simulink model "hyd_hyb_2_int_cont_Final"  (Simulink 8.2)
settings: Solver=ode4  StartTime=0  StopTime=3005  FixedStep=0.01  MaxStep=.4  RelTol=1e-8
InitFcn:
  | const_3_new
values from neighbouring files (symbols this model uses):
  Af = 6.3    [brk_enrg.m]    (also in brk_enrg_1.m)
  BSFC_906_205 = [3.5684 4.3466 5.1668 6.0769 6.988 7.8992 8.8104 9.7336 10.8548 11.9809 13.1112 14.2571 ... (663 elements, 39x17)]    [BSFC_map_906_205.mat]
  Cd = 0.55    [brk_enrg.m]    (also in brk_enrg_1.m)
  den = 1.202    [brk_enrg.m]    (also in brk_enrg_1.m)
  fr = 0.01    [brk_enrg.m]    (also in brk_enrg_1.m)
undefined symbols (not defined in the file or in its folder): clutchRise, down_spd_2, down_spd_3, down_spd_4, down_spd_c, Driving_Cycle, fuel_density, gearshift, I_wheel, Idle_spd_eng_906, M1_hydr, p_v_15, pmax_125, qv_125, Rw, sec_eng_sfc_map, T0, T1, T_max_906, T_min, TC_spd_ratio_max, teta_new_10, torque_convertor, Twait, up_spd_1, up_spd_2, up_spd_3, up_spd_c, v_p_10, v_p_15, v_p_5
libraries: neural x1742, fl_lib x43, nesl_utility x30, sdl_lib x14, simulink x4, simulink_need_slupdate x1
(part 24 of 26)

== system hyd_hyb_2_int_cont_Final/controller1/optimized controller/SOC upper 0.5/SOC upper 0.6/SOC upper 0.7/SOC upper 0.8/net_col_c_d_8_9/Layer 1/IW{1,1} ==
  "pd{1,1}" : Inport  PortDimensions=2
  "IW{1,1}(1,:)'" : Constant  Value=[5.2297082715673504;5.6273231620052648]
  "IW{1,1}(10,:)'" : Constant  Value=[5.3271967786741863;-5.5242837498455462]
  "IW{1,1}(11,:)'" : Constant  Value=[-5.7316192074747656;-5.0965749699765555]
  "IW{1,1}(12,:)'" : Constant  Value=[-6.7199302055662882;-3.6723493871487363]
  "IW{1,1}(13,:)'" : Constant  Value=[7.6310486911057183;-0.45691067438364946]
  "IW{1,1}(14,:)'" : Constant  Value=[-1.6156307363721207;-7.4985197467728266]
  "IW{1,1}(15,:)'" : Constant  Value=[7.6396721651827342;0.67767130428367428]
  "IW{1,1}(16,:)'" : Constant  Value=[-2.3794289636929844;-7.3027289928163359]
  "IW{1,1}(17,:)'" : Constant  Value=[7.609056298019194;0.96781732819446276]
  "IW{1,1}(18,:)'" : Constant  Value=[6.1297798419043019;4.6002468076239618]
  "IW{1,1}(19,:)'" : Constant  Value=[3.5487733537087367;6.8101240186103311]
  "IW{1,1}(2,:)'" : Constant  Value=[-1.7709080977346265;-7.442340947364527]
  "IW{1,1}(20,:)'" : Constant  Value=[4.6726604445306537;6.1099961278946511]
  "IW{1,1}(21,:)'" : Constant  Value=[3.625039631767633;-6.7490388004175426]
  "IW{1,1}(22,:)'" : Constant  Value=[2.3767648218081212;-7.2680324227364457]
  "IW{1,1}(23,:)'" : Constant  Value=[2.2051248172556823;7.3409202753957548]
  "IW{1,1}(24,:)'" : Constant  Value=[3.6000602042212226;6.7549906302868843]
  "IW{1,1}(25,:)'" : Constant  Value=[-6.6712233436411381;-3.6896842846457427]
  "IW{1,1}(26,:)'" : Constant  Value=[3.4549485140385632;-6.8529757203212176]
  "IW{1,1}(27,:)'" : Constant  Value=[3.9232555663050319;6.4420462296280734]
  "IW{1,1}(28,:)'" : Constant  Value=[0.80122508503254797;7.778785998543821]
  "IW{1,1}(29,:)'" : Constant  Value=[-3.0811819967324192;-6.8692043192527965]
  "IW{1,1}(3,:)'" : Constant  Value=[3.9369646308008228;6.5356049546767476]
  "IW{1,1}(30,:)'" : Constant  Value=[7.6499292380272141;1.3230721920060999]
  "IW{1,1}(4,:)'" : Constant  Value=[3.2253351379319164;6.9688557463217036]
  "IW{1,1}(5,:)'" : Constant  Value=[3.9082074631794095;6.5873222203975601]
  "IW{1,1}(6,:)'" : Constant  Value=[7.2679721529349646;2.4081951987663022]
  "IW{1,1}(7,:)'" : Constant  Value=[-7.5805190406682321;-1.0513803544595217]
  "IW{1,1}(8,:)'" : Constant  Value=[-3.9971056760000749;-6.5538153054232726]
  "IW{1,1}(9,:)'" : Constant  Value=[-5.1483853775004791;-5.691072714021133]
  Mux : Mux  Inputs=30
  dotprod{1..30} (30 alike) : neural/Weight Functions/dotprod
  "iz{1,1}" : Outport
  wires:
  Mux/1 -> "iz{1,1}"/1
  dotprod30/1 -> Mux/30
  "IW{1,1}(30,:)'"/1 -> dotprod30/1
  dotprod29/1 -> Mux/29
  "IW{1,1}(29,:)'"/1 -> dotprod29/1
  dotprod28/1 -> Mux/28
  "IW{1,1}(28,:)'"/1 -> dotprod28/1
  dotprod27/1 -> Mux/27
  "IW{1,1}(27,:)'"/1 -> dotprod27/1
  dotprod26/1 -> Mux/26
  "IW{1,1}(26,:)'"/1 -> dotprod26/1
  dotprod25/1 -> Mux/25
  "IW{1,1}(25,:)'"/1 -> dotprod25/1
  dotprod24/1 -> Mux/24
  "IW{1,1}(24,:)'"/1 -> dotprod24/1
  dotprod23/1 -> Mux/23
  "IW{1,1}(23,:)'"/1 -> dotprod23/1
  dotprod22/1 -> Mux/22
  "IW{1,1}(22,:)'"/1 -> dotprod22/1
  dotprod21/1 -> Mux/21
  "IW{1,1}(21,:)'"/1 -> dotprod21/1
  dotprod20/1 -> Mux/20
  "IW{1,1}(20,:)'"/1 -> dotprod20/1
  dotprod19/1 -> Mux/19
  "IW{1,1}(19,:)'"/1 -> dotprod19/1
  dotprod18/1 -> Mux/18
  "IW{1,1}(18,:)'"/1 -> dotprod18/1
  dotprod17/1 -> Mux/17
  "IW{1,1}(17,:)'"/1 -> dotprod17/1
  dotprod16/1 -> Mux/16
  "IW{1,1}(16,:)'"/1 -> dotprod16/1
  dotprod15/1 -> Mux/15
  "IW{1,1}(15,:)'"/1 -> dotprod15/1
  dotprod14/1 -> Mux/14
  "IW{1,1}(14,:)'"/1 -> dotprod14/1
  dotprod13/1 -> Mux/13
  "IW{1,1}(13,:)'"/1 -> dotprod13/1
  dotprod12/1 -> Mux/12
  "IW{1,1}(12,:)'"/1 -> dotprod12/1
  dotprod11/1 -> Mux/11
  "IW{1,1}(11,:)'"/1 -> dotprod11/1
  dotprod10/1 -> Mux/10
  "IW{1,1}(10,:)'"/1 -> dotprod10/1
  dotprod9/1 -> Mux/9
  "IW{1,1}(9,:)'"/1 -> dotprod9/1
  dotprod8/1 -> Mux/8
  "IW{1,1}(8,:)'"/1 -> dotprod8/1
  dotprod7/1 -> Mux/7
  "IW{1,1}(7,:)'"/1 -> dotprod7/1
  dotprod6/1 -> Mux/6
  "IW{1,1}(6,:)'"/1 -> dotprod6/1
  dotprod5/1 -> Mux/5
  "IW{1,1}(5,:)'"/1 -> dotprod5/1
  dotprod4/1 -> Mux/4
  "IW{1,1}(4,:)'"/1 -> dotprod4/1
  dotprod3/1 -> Mux/3
  "IW{1,1}(3,:)'"/1 -> dotprod3/1
  dotprod2/1 -> Mux/2
  "IW{1,1}(2,:)'"/1 -> dotprod2/1
  dotprod1/1 -> Mux/1
  "pd{1,1}"/1 -> dotprod30/2, dotprod29/2, dotprod28/2, dotprod27/2, dotprod26/2, dotprod25/2, dotprod24/2, dotprod23/2, dotprod22/2, dotprod21/2, dotprod20/2, dotprod19/2, dotprod18/2, dotprod17/2, dotprod16/2, dotprod15/2, dotprod14/2, dotprod13/2, dotprod12/2, dotprod11/2, dotprod10/2, dotprod9/2, dotprod8/2, dotprod7/2, dotprod6/2, dotprod5/2, dotprod4/2, dotprod3/2, dotprod2/2, dotprod1/2
  "IW{1,1}(1,:)'"/1 -> dotprod1/1

== system hyd_hyb_2_int_cont_Final/controller1/optimized controller/SOC upper 0.5/SOC upper 0.6/SOC upper 0.7/SOC upper 0.8/net_col_c_d_8_9/Layer 2/Delays 1 ==
  "p{2}" : Inport  PortDimensions=30
  mux : Mux  Inputs=1
  "pd{2,1}" : Outport
  wires:
  mux/1 -> "pd{2,1}"/1
  "p{2}"/1 -> mux/1

== system hyd_hyb_2_int_cont_Final/controller1/optimized controller/SOC upper 0.5/SOC upper 0.6/SOC upper 0.7/SOC upper 0.8/net_col_c_d_8_9/Layer 2/LW{2,1} ==
  "ad{2,1}" : Inport  PortDimensions=30
  "IW{2,1}(1,:)'" : Constant  Value=[-0.01337138047549283;-0.28095158446727192;-0.16503164756388625;-0.45784461439440827;-0.12950501000005665;0.18202533973662072;0.016691236840415163;-0.14736753510045073;-0.38808878997216451;0.30255086537017006;0.07200208164381916;0.56168796965376189;-0.45033706536037649;0.28342366252104456;-0.17290280054727319;0.099768076125372654;-0.30844788844149273;-0.48874450861518076;-0.095930800808782177;-0.085620551553359056;0.18719700480212248;0.20192166498704908;-0.39439281517504299;-0.1761066303970199;-0.27960083721330503;0.11415904568162979;0.33813666987772623;0.071160346914529549;-0.47467652276569738;0.53680426915168111]
  "IW{2,1}(10,:)'" : Constant  Value=[-0.12877936609158763;-0.47587728279057023;0.1877867845721852;-0.084215930155876292;-0.20839808710547195;-0.13666953154125866;0.35591088137150056;-0.14007053087915702;0.51663619503232094;0.44705116455638544;-0.20614768887343585;-0.30817662964547182;-0.11375336795447927;0.077503999867870141;-0.23895377418591321;-0.0041563317406688822;-0.35865623913112427;0.25243705879368766;-0.52549121959207545;-0.42448219196266607;0.39264365797558393;0.27932335621641147;-0.36925219355094963;0.31565733162137832;0.20118306741746081;-0.25536563672747148;0.14832240983231315;0.066442949083321184;-0.071777147677271794;-0.42005348211208249]
  "IW{2,1}(11,:)'" : Constant  Value=[0.42887485853389118;-0.48701290610635062;-0.018546953988905174;0.15083692230155854;-0.41499077481347629;-0.21432733820014618;-0.012686165000563823;0.42509965196917981;-0.035819058983909802;-0.57481434848859814;0.19499799217111058;0.15568572289966565;-0.18305925453768279;-0.021450482313967071;0.3661066323547566;0.046817351945665463;-0.35615081739053278;-0.0063144505914314491;0.47626161010990564;0.39519202026262112;0.38413528174445222;0.3325880859338356;0.31746601920344364;0.14701202960728005;0.31657075402271662;0.24974972097089457;0.37299354569369358;0.084383088674610862;0.12045514477163605;0.2263767581285841]
  "IW{2,1}(12,:)'" : Constant  Value=[-0.44785493325983433;0.29952879966428503;-0.3588623235389265;-0.18458233023437801;0.49357052273034574;-0.13165235315396617;-0.10119602952912031;-0.10260838617534325;-0.17126538459857643;-0.30572828086222886;0.29790579152294422;0.19409119242637829;0.21566604834666511;0.33688116278072733;0.24763106757804323;0.078656751347893794;-0.43440903548495796;-0.45551268819722224;0.38969396678151003;-0.22465887258290596;-0.23546967211109304;-0.29929980636648901;0.22900416155132622;0.092413420687598224;0.48574420859216094;-0.22374516140450662;-0.083901963510923591;0.30886163712497755;0.21685949872336133;0.061952852103937785]
  "IW{2,1}(13,:)'" : Constant  Value=[-0.31418908401409446;-0.26007649238943248;0.31954309252078866;-0.16814071124454713;-0.15763410114005866;-0.10401807888790811;-0.46102846038269585;0.25271545605528017;0.01007848864071678;-0.10314792312684756;0.1726838125829338;0.36931842608368276;0.3301744921687324;-0.3439717376221833;-0.2931194999336918;0.1567186462139446;0.028852670221030441;0.38095801360245324;-0.023951265973831792;-0.32362259435845647;0.1213573066251033;0.32671598025856813;-0.35992893349504707;0.39909077457579401;-0.31688075594830212;-0.26439448936765109;0.37925680164647591;0.40562213625379306;0.37358297909075522;-0.42747484886868137]
  "IW{2,1}(14,:)'" : Constant  Value=[0.44783714821849963;0.21410181269156028;0.0017982430301030691;-0.19465254425693904;-0.18537384377184216;0.56490668359860297;-0.14690102947081646;0.076463921210399077;-0.16204433876665503;0.36350674442905334;0.16992392694215283;0.12886172891572309;0.23470151490794303;-0.070262818563302507;0.15277790832690061;0.3242695891352198;-0.33513718132499548;0.02823581430237003;0.24246033346808166;-0.42088994103419702;-0.17302374067804713;0.0073299722701979375;0.12968092832442085;-0.17307640423438062;-0.47559342269963734;0.095925192804616047;-0.13976047960361213;0.1571766674662837;-0.50441234690224679;-0.52416221892977011]
  "IW{2,1}(15,:)'" : Constant  Value=[0.26248732607376118;0.49532186242617754;-0.50454391880052862;-0.327207659699144;-0.43642565615523787;-0.14607435486446912;0.40130138540730037;0.31215082826881574;0.25486274803394454;0.60973007559694337;0.33833680853014564;-0.52453062690783414;0.39088455441145586;0.078339660177359341;0.40661236585034116;-0.35387516353774034;0.0016044841618512832;0.16386400331983944;0.19567426275447886;-0.12013064942167608;-0.31208369937469305;-0.0072081351890981192;-0.089588039665270916;0.11873875205253952;-0.27994249441980767;-0.13508489135594531;0.17255143878117848;-0.22581311631817616;-0.12644715914540158;-0.087171365990115116]
  "IW{2,1}(16,:)'" : Constant  Value=[0.25849307971468227;-0.081086656772899016;-0.37114809548005617;0.25244334293572629;-0.43907061163932803;0.095907918504148287;0.00087443781706484985;0.0071769632098506201;-0.11045664266875481;0.27238467563200114;-0.48182337479969028;0.076178929039177418;-0.4290672354726795;0.1644471337080444;0.35539205679760533;-0.074161740982161509;-0.51362051686285326;-0.34302321993807111;0.093099865710912874;0.012061499461902237;-0.47011394461600625;0.082969559697853607;0.0082701803952539496;-0.18642695085794539;0.22494168965042269;0.38183906703217679;-0.2935199001717782;-0.42174419286554787;-0.096451078485828387;0.40643207224803157]
  "IW{2,1}(17,:)'" : Constant  Value=[-0.10985208829065081;0.20287921542786699;0.1385279804468377;-0.076191504229959808;-0.42580080975566248;0.14817967802448828;0.11089975305435197;0.42803122009154243;-0.37393350163109551;0.31184811677206176;0.19699926242620167;0.52047209393507121;0.23701277003839935;0.1655843122380026;0.30175170983751803;0.17624100149760077;0.16361599905038912;0.18855720151875785;-0.1980741670478727;-0.32967865622549619;-0.38664710435007577;-0.22380162289117694;-0.39779045097547805;0.42249107453632723;0.27410450945606801;0.34088477559968205;-0.047198280755287619;-0.21191075972781317;-0.25376453847567082;0.43719807532785637]
  "IW{2,1}(18,:)'" : Constant  Value=[0.36313113458044954;-0.45746696787424895;-0.34426640866793873;-0.32170606512569289;0.42057890979287332;-0.00181978915271525;0.1459272658151563;0.18519960726847709;-0.16106364805954584;-0.39963178414914424;-0.22157734573905408;0.32219734224641583;0.20062914162945403;-0.2545292998498267;0.35935237519802937;0.012926126328639867;0.45577500604689425;0.36355616414433117;0.43178218463070439;0.34368428016565061;-0.31142493031492391;0.0042379127935098272;0.13340593049872332;-0.08845582234622143;0.18892338612544646;0.15198499384350672;0.45809972028106005;0.0018658778608795163;0.15039472963027983;0.30140556377514649]
  "IW{2,1}(19,:)'" : Constant  Value=[-0.40024936770151809;-0.069990039918450486;-0.26846229603419031;-0.26796866623906085;0.14370094057409916;-0.13257757022718608;-0.14202670147981977;-0.11555052588655544;0.482513279982757;0.37540224984567433;0.045720880165311013;-0.34880970877999468;-0.084645593633637439;0.19675127038319284;0.3418468810673268;0.35818859368575673;0.28623906243260938;0.054468861071998345;-0.27715664772524884;0.53345353050796507;-0.28015882124595443;-0.22544662860211423;-0.18490067544779457;0.050219360778613213;-0.19199718879623881;0.35888889470113017;0.66475560302036896;0.36863432937801865;-0.18167039999527965;-0.24167470599647797]
  "IW{2,1}(2,:)'" : Constant  Value=[-0.17215825353448597;0.18276874727348558;0.41829311891188098;-0.38319630265046389;-0.3461732726853971;-0.34806187602749161;-0.031378949842030157;-0.053730269792174441;-0.31708091642943365;0.075250731893123868;0.077395970639861186;-0.43108799199953118;0.43648394912194644;0.23844679788483208;0.036329127847019096;-0.42482570873919556;0.12541331002972139;0.23262681737061769;-0.0884879688988226;-0.47080458980419865;-0.40740713775100956;0.29880858504804658;0.091433884817461827;0.27874073282329404;0.10002048156338145;0.31048702807117606;-0.40704393944417033;-0.32206176394111002;-0.20514600682087514;0.024424815321697994]
  "IW{2,1}(20,:)'" : Constant  Value=[-0.38223287733513139;-0.11651569769184145;-0.23275015969836332;-0.45779281349779999;0.18066173843842123;0.023085666550045913;-0.40820570256541683;0.33916201754344916;-0.11266284908532383;-0.16903683306578501;-0.28648097306394582;-0.43083926662310867;-0.46970003759028961;0.41457450668029128;0.31816631920923794;-0.071101200865994502;-0.37495314507762695;-0.33674199314348485;0.25952681605999778;0.23489594693223437;-0.10125495737454836;0.2101344479027816;0.37005895040677289;0.30587065555411441;0.063143632678687708;0.28455037362744107;0.36363792391389332;0.20145534806805193;0.41971752395757178;-0.079369589634068052]
  "IW{2,1}(21,:)'" : Constant  Value=[-0.44587557795505756;0.32740561952944419;0.38242609904269403;0.37430642058075175;-0.16068302641590787;0.41726742666478989;0.14942045232082238;-0.1621253464371438;-0.32622675546004437;-0.32116770641464681;-0.36557171156205387;0.36502044171332571;0.27334850926184612;-0.30009388144256499;0.42802284457067563;0.14466585140373142;-0.060258875798323314;-0.41742951301170372;0.23808745747733381;0.18585314943781042;0.053722779449327886;0.054664173200892778;0.15483250040667215;0.20287679547981879;0.38366880349904847;0.20457898436260571;0.16469380057399624;-0.29360888772298599;-0.42080913578445506;0.046179995566540122]
  "IW{2,1}(22,:)'" : Constant  Value=[0.21636058009297521;-0.048628316899150946;0.22400575098582581;-0.16240083162601937;-0.27981474426276076;-0.07157564563365007;-0.2350472772516605;0.25118377072926423;0.35912589234946107;0.076186507209085083;0.22161975625797509;0.15702030333433434;-0.43095922425841232;-0.4152102657603447;-0.43862743602039422;-0.011235991663650854;-0.13312099176855877;0.30415086968488675;-0.31121424612693388;-0.33791185979529931;0.23077084628641112;0.28344905486157063;-0.53611342527279215;-0.2015566312576936;-0.21547089435873504;0.39763390440517432;-0.16950914148141671;-0.53712866466562004;-0.17652712530811226;-0.3427999056643391]
  "IW{2,1}(23,:)'" : Constant  Value=[-0.35280675392156435;-0.3010673935021328;0.41608246319314468;-0.33849225058032895;0.22991102374993189;0.32333061389512163;-0.084652038040488695;-0.19154035498842203;0.29772109061750851;0.30170392247270678;0.3581450372963832;0.065280684788798629;0.2767167597231473;-0.20308742181054668;-0.44195273570782612;-0.3732427508820168;-0.22105404763754652;-0.10469193681428836;0.4311958385750429;-0.065795408024307694;-0.15641781925152709;-0.23510602786800178;0.30249970235825796;0.22936052939810028;-0.39549613705286923;-0.3361265711189701;-0.16519320632831874;-0.26305919328914285;-0.32180519874075603;0.35878969944792594]
  "IW{2,1}(24,:)'" : Constant  Value=[-0.39954818514968038;-0.38584858299109431;-0.07541952652740487;-0.20450550652773936;-0.0093294507875483438;-0.52669564687724446;0.38351113947591614;0.49383839797094709;-0.18039270622145775;-0.29122897578217299;-0.35920060664312431;0.14092558998120627;0.1980150762491856;-0.047907822931633183;0.34783764602231987;-0.64517520829618358;-0.2143138418484537;0.081914435692262089;-0.29039775640602383;0.30932947623581064;-0.38977163386739161;0.2512912654662966;0.2307235760701683;-0.043076335891067401;0.23872064932855175;-0.33349036996482201;0.069572227976522599;-0.55478052347580242;0.57110817405267611;-0.093336083351195434]
  "IW{2,1}(25,:)'" : Constant  Value=[-0.36763713801641079;0.34825941736863519;0.42454373002714263;0.28313626181003215;0.10629586035838771;0.34705077686493213;-0.17379537371878279;0.3939219596097247;-0.35511501178728516;0.30538906314992975;-0.33086578883535178;0.27933314751540111;0.063771123735152049;0.078970554978038288;0.37006133520646994;0.11259355433337212;0.35343274160777882;-0.28812607166442028;0.16935010416359675;-0.36502314661876956;0.4617288314214128;-0.11547186509230255;0.046403829322165462;-0.22169916114863508;0.38623192167903392;0.41959430731705616;0.32414954279425734;-0.075205581037819505;0.15790599393630386;0.37414078448769206]
  "IW{2,1}(26,:)'" : Constant  Value=[0.52573288749680702;0.40034099811987017;-0.26614507154943695;-0.17639794797590561;-0.16509663241579434;-0.22664989154653412;0.065061930792583406;0.11228960496979679;-0.01586496866196091;-0.16684352947742317;0.20796323056056001;0.54615267784543953;-0.23128711278068634;0.15776886108586116;-0.44292144158175684;-0.097466048631904056;-0.31799965938536556;-0.26010448981072015;-0.17307094257448311;-0.18913055968361217;0.017575167502147836;-0.041939063149283952;0.43861409427711379;0.013801766692959388;-0.22718167304398099;-0.28560079969741436;0.38903185419408859;-0.50312163030440182;0.31408250210754701;0.37665101738300977]
  "IW{2,1}(27,:)'" : Constant  Value=[0.33171371527714699;0.16094842839367779;-0.43394200050156834;0.22369320776146284;0.29166008248048902;0.27252752447324446;0.36954493029020469;0.51971771989356952;0.18853850210773501;-0.38736530853307249;0.20057642766429876;-0.16322009210808275;-0.46668975066387747;0.12815905353447782;0.41584758680762668;-0.15897244145771519;0.0075665170752451686;0.29045355417878171;-0.30879748700008658;-0.52223839170982966;0.200570563279833;0.10492517778771469;-0.28682697922584538;-0.2809972048979455;-0.082528614229641278;-0.099363495498231716;-0.18145867697150497;0.31196931752430912;-0.24493689473639332;-0.052841565698375143]
  "IW{2,1}(28,:)'" : Constant  Value=[0.46352443075216065;-0.16020812737041185;0.11617096384756628;0.084739151585717598;-0.005397449191996649;0.33740212936135172;0.15352153436759949;-0.37872991144121126;0.44672032463976857;-0.21011996332232627;-0.24880878776884566;0.43728779774751936;-0.33719912988739931;-0.23352942228598422;-0.15288243110157007;-0.16213244976095589;-0.14952286234315387;0.087128460914169911;-0.33304589754894048;0.58262554536069033;-0.31376856708129131;0.10334800924732476;-0.3263613131405364;0.18621928005460742;0.26070946741513235;0.37499179915623981;0.32227956879442249;0.16628976408850452;0.36124072198989432;0.30241654834024695]
  "IW{2,1}(29,:)'" : Constant  Value=[-0.032135656874180109;0.07782054152925845;0.0040382908002594654;0.29595481169961307;-0.49719562651437715;0.045881703436677357;-0.13674251619170574;-0.3651454127633163;0.37753762710669941;0.015070789295483392;0.38137989535205796;-0.44740028262003767;-0.35796445021792894;0.16308738337540649;0.40614755086184079;0.25417112757858445;0.14995071389086537;0.15778841738949609;-0.42509024816716812;-0.35724418187985457;-0.34910295369786914;0.15678899210307395;0.3638484253106663;-0.47125321250771501;0.091804607727718243;-0.16270328791294161;-0.37000259210045022;-0.38839262070853597;0.010645208949013392;0.28440502208264956]
  "IW{2,1}(3,:)'" : Constant  Value=[0.49589068496557848;-0.099790505715858333;0.19907432476762735;-0.15103188678785306;-0.12154785305984357;0.019985691440159107;0.42440771674479172;-0.11330245780436633;-0.098572061777852077;0.14407479352187666;-0.36614585708981523;-0.31411433621055823;-0.19653030232966009;-0.093984011944081;-0.2498301487471056;0.17850968751630122;0.23507025422671757;0.25555893873650432;0.47760052403438508;0.49303832040789719;0.18479749666760689;0.54780287375494663;-0.024168247943590095;-0.049713587351482194;-0.052804916716366966;-0.5531654257761387;-0.042124019466908975;0.23243801723715074;0.085949288304206062;0.50513626708486281]
  "IW{2,1}(30,:)'" : Constant  Value=[-0.049539611263283823;-0.21050388986124069;0.36854535771673841;0.35646862647244404;-0.12945675563556919;-0.058142221328256034;-0.35472560017380977;-0.22294006236398664;0.36491124821386312;-0.37704006333052648;0.15195308817791128;-0.23083299918527303;-0.49723252321599637;-0.15776468530387094;0.29131945332116121;-0.4919654897132395;-0.22849123180584444;-0.40567867617927333;0.16937452809726758;0.2277476637397505;-0.29036301627548894;-0.34298893911860306;0.28254362300492175;0.13584255131354611;-0.3009081560459887;-0.007315560129343153;0.22990789594098793;0.35945961483827538;-0.321277457766523;0.34274055153256355]
  "IW{2,1}(31,:)'" : Constant  Value=[-0.16132811963159346;-0.05062360531953828;-0.37672644648510456;0.067530469560452125;-0.12358081954064448;-0.3073367745663908;-0.49757470974951779;-0.035677851183680019;-0.23072579152072942;0.31870379457497505;-0.20214077549455436;-0.28618563654097257;-0.096067278036762557;0.46270416622365801;0.46748405885863137;-0.16688562101496926;-0.34790847357964105;0.035411119946928866;-0.30970842080054145;0.4166094000270677;-0.094592761732787842;-0.17090119044849839;0.4591296289596577;-0.22987076579145688;0.049029546631407489;0.20057854380811307;-0.43708930157420478;0.16332184135462674;-0.24965469474306659;-0.4399386232667104]
  "IW{2,1}(32,:)'" : Constant  Value=[-0.10960003224877882;-0.43018847706807839;0.51600023685217689;-0.54680117952894602;-0.20074674176317087;0.24530234075343244;0.56756028812749448;0.43984120340234445;-0.36682999450401838;-0.31524978946179366;-0.44416640904854154;0.042777969880379386;0.19299135061331887;0.0085978860053103744;0.10492200544185569;0.013562235105007201;0.0067268931617746946;0.41604794698378683;0.061651283693760474;0.080303691432675309;0.13375639018360874;0.45708453079471084;-0.01589778034387028;0.16772634511867013;-0.10718683962112731;-0.073499940581839965;-0.11748968833344255;0.31257620440872097;-0.44650296770344555;-0.24283220910008219]
  "IW{2,1}(33,:)'" : Constant  Value=[0.44309314489416107;-0.19407213446434163;0.29095073825095674;0.41485201784327885;0.1997842537710604;-0.048894504535411817;0.1483106326562916;-0.030054084121407171;0.47059399352590481;-0.039251170687077938;-0.27095604380657484;-0.018301125390313259;-0.22525355966166052;0.18209500442869841;0.044678593285385641;0.41350426852397471;-0.42466178548153199;0.25563245497413783;-0.31647268041785948;-0.29381900366836344;-0.17082615688039818;-0.36473588127055045;0.54568761453444214;0.33891407074749547;0.432181267674211;0.014859918413714958;-0.22028136579632701;-0.0023456653160113861;0.51817674045931039;0.15125382899578843]
  "IW{2,1}(34,:)'" : Constant  Value=[0.32921363085196775;0.05562151583568159;-0.35034077400782743;0.25012478306330471;-0.13017943304241886;0.3433967030031615;0.29597295356986908;-0.210137558377266;0.41214383333754445;-0.21845816248736727;-0.29589408914469384;-0.3303403345752412;-0.2198668799882193;0.37805878861588205;-0.344667271778625;-0.1090280719538483;-0.096313448723471529;-0.26228271369138578;-0.40027321789097597;0.42086673720411261;-0.12071877246969784;0.046042297244496162;0.34950811699336254;0.47448331798639004;-0.16177072531830192;-0.33548521113654028;0.36399399605948313;0.4851527629749392;-0.42119637494713347;0.20255457814559419]
  "IW{2,1}(35,:)'" : Constant  Value=[-0.095304181568827057;0.2411861797336044;0.38093256060531172;-0.38482836195195164;-0.20955113698622385;-0.22805076013641554;0.29720949253117951;-0.16063823229995752;0.35958482194483726;-0.026755554233294628;0.15727655096687126;-0.1728035938490618;0.057094024908256977;0.01526672348094682;0.39237780589301491;0.45867076500022103;0.5581416472088867;0.42758505831315785;-0.030390232255899031;0.073219907667348982;0.16574749841546035;-0.0048104100066032243;0.1788932676861425;-0.35448965871809562;0.55469357014382281;-0.56191267035479397;0.1111925277258709;0.13606601060132853;-0.12582903254498432;-0.21658224463438697]
  "IW{2,1}(36,:)'" : Constant  Value=[-0.19128044878020015;-0.10994557683321811;-0.49575647432059594;-0.52362892158725849;-0.27280257170184113;0.068185085406951021;-0.19714897729908581;0.35444168343320737;-0.092621955922172955;-0.49572669586490964;0.57202494584954167;0.3278340339248309;-0.50884757125464375;-0.27301784455461925;0.14507662918967204;-0.27534742727516476;0.025149085320547541;-0.20293411172988976;0.1312925370460527;-0.19007693669979023;0.052619675958508853;-0.44475110339492713;0.045983399704365359;-0.14992425385717129;-0.41466020405617054;0.41639532250839117;0.29279888946762456;0.43706899341141237;-0.23911442125931215;-0.46610174086974565]
  "IW{2,1}(37,:)'" : Constant  Value=[0.23372418297866729;0.053635735470619075;0.42145802794127607;0.47036015295360345;-0.016586558717063344;-0.32643857468136195;-0.28371518742311513;0.09803946857466575;0.32359913792801265;-0.13943681923849011;0.2984112743599634;0.38504949535570676;-0.46419048466057555;0.35449184941958323;-0.45034003692534913;0.007248493685549617;0.41318157774100067;0.13694508099330388;-0.14105313192375307;0.31040845146413543;-0.42577850854320587;-0.39614305903626607;0.036802040775937885;-0.28240306172789981;0.34335509546632009;-0.11303859296920049;0.083892521426806671;-0.33789689302338088;-0.099731721936320822;0.11018262070533315]
  "IW{2,1}(38,:)'" : Constant  Value=[0.28099261784900359;0.3193879716122931;0.42728098016589555;0.31657025567995195;0.45108980800229204;0.22831118471030978;-0.13386410394994516;-0.068164403512579047;-0.34508904764661219;0.3876237504787986;-0.00044624195542457989;0.16554559092654872;0.23283464736276793;0.36393882914020215;0.36640897303212555;0.013768397221129993;0.41075269006827014;0.13356036927354209;-0.28997312141977305;0.073751840513592556;-0.33401994822798786;0.30757744605086701;-0.40284577898625334;0.072202088999151884;-0.4171213915393871;-0.12573436898940651;0.0068675004406296737;-0.38796886773544875;-0.38360973643403273;-0.19326434765954589]
  "IW{2,1}(39,:)'" : Constant  Value=[-0.32757754884726292;-0.079798672827026032;-0.43617646227829049;0.092408938920207837;-0.18053063251777915;-0.45222968309602551;-0.033681065820181343;0.09233311332115815;0.36045287074028109;0.18767183113811103;0.41516942119227845;-0.30722382070363563;-0.4254720917525931;0.19297915653605641;0.39811802646308864;-0.33799835929339955;0.26481767727562383;-0.07583865459147382;0.052761978622893169;-0.41484250073497653;0.46060901006667493;-0.17291735604678432;0.23866041452916714;-0.43666657192707836;0.11272059076303981;0.4282678664838101;-0.2013228359819747;-0.33541571927699376;-0.23190326147435741;-0.28162051653985287]
  "IW{2,1}(4,:)'" : Constant  Value=[-0.1033101588955887;0.19723778811968759;-0.050334669662173023;-0.40401992912827744;-0.37203771263235458;-0.070862259775875375;0.17265165146385897;0.45120564616098313;-0.30033568297024749;-0.095377549075230869;-0.22461822793898964;-0.033382595978892565;0.051799243492291397;-0.1920663496419826;0.44772114437237798;-0.20290977837278368;-0.45208788758642804;0.0041700277232766952;-0.32896667827504528;-0.44277943415629684;-0.16884441208067191;-0.15018007843166128;-0.35614725409236908;0.061998033725852567;0.4472656016464307;0.42130255096292724;0.3946318694739227;0.30959329779026257;0.40045309040204125;0.030639466028702874]
  "IW{2,1}(40,:)'" : Constant  Value=[0.15046878531670518;-0.30672503393827633;0.22411832901650924;0.13509624688313518;-0.34571378382937207;0.066805973069938129;-0.27876460666036157;0.46102713903022396;-0.25291888010956842;0.10868076501566555;0.25246055232063602;0.17258627267115154;0.24430979399509889;0.089281500966414032;0.33788350015495006;0.017431540868197235;0.44545920044149367;-0.39497816501439265;-0.1144001399018838;0.31038743348810499;0.19121596309155492;0.0080988710505405168;-0.21618039945702153;0.46885068859535084;-0.29164901874853866;0.4655136896867117;-0.32013789260363212;0.0074623519291403704;0.43115342101542409;0.45197306786998637]
  "IW{2,1}(5,:)'" : Constant  Value=[0.035084508806841483;-0.22309699429840305;0.31847817403339324;0.075239299837429094;-0.39273716495940869;-0.094184962576489561;-0.033172473093734313;0.14606226763656099;0.0930816854706535;-0.43223819820786291;-0.23023870285717199;-0.46103740043144392;0.33041911494577042;-0.0038860200166226889;0.27567793872830865;-0.43963490714533127;-0.21732527501532825;-0.15757997026674148;-0.40296802299020507;0.11323597593401873;0.39098520712327417;0.18849632930202284;0.40028433685325543;0.43204735194293514;-0.45141872795683829;0.27813157442337627;0.47632451016231397;-0.33572133057980974;-0.40728861097546198;0.1821846099423006]
  "IW{2,1}(6,:)'" : Constant  Value=[0.061689139330504961;0.47503152929291875;-0.23508033613305421;0.032368945162306394;0.16141041481701496;0.49898938245359176;0.14620097648708399;-0.12998956897472833;0.26981476837151974;-0.14479328909394082;0.37118496890031782;0.12247390959540533;0.60256439895707281;0.2732823395600209;0.27706091645880071;-0.24813973636499584;-0.37723372169828717;0.031282335938951286;-0.16495803738202042;0.19539376318442231;0.22644918670236683;-0.018018305447286539;-0.43812820063951885;-0.039801640209229799;-0.42404653533843284;-0.1150955597325749;-0.20902331603204333;-0.44516744448648798;-0.3109361036481984;0.26913433021580241]
  "IW{2,1}(7,:)'" : Constant  Value=[0.37549651462473788;0.20016705528187573;-0.20630460323959807;0.18473032347994298;0.30139670694994908;-0.32882887048936998;0.034469628218871291;0.062888103668764933;-0.42373630734630624;-0.2026860520356113;0.45737971815981304;0.27491666965410916;-0.28601117658794017;-0.22258265729116961;0.44516348538260619;-0.20008300765465481;-0.17685032666878078;0.095713508905817923;-0.44745074901871257;-0.29721183143062513;-0.38889753890692025;0.082991607687713173;0.41465796413739264;0.27770788778360733;0.33246673320645831;0.13176507381700622;0.06853705330887773;-0.16090863406100647;-0.49708819367776025;0.12290505058921722]
  "IW{2,1}(8,:)'" : Constant  Value=[0.12895028439581618;-0.0010177320513798951;-0.13629719225032341;-0.45165414971870965;0.44758354424095537;-0.40686506362381736;-0.26955513540494597;-0.44442908676720144;0.18485782026388561;0.15019243336851781;0.19933474473485449;-0.014863908837363507;0.30239437021814047;-0.10137091311622576;-0.1207035912245293;0.11605085175893905;-0.30164213974845211;-0.22280866074564185;-0.19505302686720979;0.23219967640280631;-0.4698159463542313;0.081861226183918875;0.12039789510468725;0.42129998556648551;-0.35156531504035232;-0.18789588586684891;0.1871546109807222;-0.44837952067230014;0.44141433402483332;0.32048534399380912]
  "IW{2,1}(9,:)'" : Constant  Value=[0.093949687257767367;0.28291752064807069;-0.37801438477294214;0.38400904730423085;-0.40277799298334105;-0.17893428464271008;-0.12545782038178244;-0.30965344807437317;-0.31078103980540567;-0.07348897089833635;0.37256928599431838;-0.16735615211311111;0.27169321886679421;0.32805839937562098;-0.0051331807985233752;-0.3253297505738878;0.3002643609297499;-0.23585187783813935;-0.52318354831089209;-0.28846738635763242;-0.26888748279035318;-0.10928234646665251;-0.56936096690595006;0.19762261966641231;0.014523717854880866;-0.196534962868882;0.45761981386523953;0.090252012488458586;0.12102086920512532;-0.29466926370148916]
  Mux : Mux  Inputs=40
  dotprod{1..40} (40 alike) : neural/Weight Functions/dotprod
  "lz{2,1}" : Outport
  wires:
  Mux/1 -> "lz{2,1}"/1
  dotprod40/1 -> Mux/40
  "IW{2,1}(40,:)'"/1 -> dotprod40/1
  dotprod39/1 -> Mux/39
  "IW{2,1}(39,:)'"/1 -> dotprod39/1
  dotprod38/1 -> Mux/38
  "IW{2,1}(38,:)'"/1 -> dotprod38/1
  dotprod37/1 -> Mux/37
  "IW{2,1}(37,:)'"/1 -> dotprod37/1
  dotprod36/1 -> Mux/36
  "IW{2,1}(36,:)'"/1 -> dotprod36/1
  dotprod35/1 -> Mux/35
  "IW{2,1}(35,:)'"/1 -> dotprod35/1
  dotprod34/1 -> Mux/34
  "IW{2,1}(34,:)'"/1 -> dotprod34/1
  dotprod33/1 -> Mux/33
  "IW{2,1}(33,:)'"/1 -> dotprod33/1
  dotprod32/1 -> Mux/32
  "IW{2,1}(32,:)'"/1 -> dotprod32/1
  dotprod31/1 -> Mux/31
  "IW{2,1}(31,:)'"/1 -> dotprod31/1
  dotprod30/1 -> Mux/30
  "IW{2,1}(30,:)'"/1 -> dotprod30/1
  dotprod29/1 -> Mux/29
  "IW{2,1}(29,:)'"/1 -> dotprod29/1
  dotprod28/1 -> Mux/28
  "IW{2,1}(28,:)'"/1 -> dotprod28/1
  dotprod27/1 -> Mux/27
  "IW{2,1}(27,:)'"/1 -> dotprod27/1
  dotprod26/1 -> Mux/26
  "IW{2,1}(26,:)'"/1 -> dotprod26/1
  dotprod25/1 -> Mux/25
  "IW{2,1}(25,:)'"/1 -> dotprod25/1
  dotprod24/1 -> Mux/24
  "IW{2,1}(24,:)'"/1 -> dotprod24/1
  dotprod23/1 -> Mux/23
  "IW{2,1}(23,:)'"/1 -> dotprod23/1
  dotprod22/1 -> Mux/22
  "IW{2,1}(22,:)'"/1 -> dotprod22/1
  dotprod21/1 -> Mux/21
  "IW{2,1}(21,:)'"/1 -> dotprod21/1
  dotprod20/1 -> Mux/20
  "IW{2,1}(20,:)'"/1 -> dotprod20/1
  dotprod19/1 -> Mux/19
  "IW{2,1}(19,:)'"/1 -> dotprod19/1
  dotprod18/1 -> Mux/18
  "IW{2,1}(18,:)'"/1 -> dotprod18/1
  dotprod17/1 -> Mux/17
  "IW{2,1}(17,:)'"/1 -> dotprod17/1
  dotprod16/1 -> Mux/16
  "IW{2,1}(16,:)'"/1 -> dotprod16/1
  dotprod15/1 -> Mux/15
  "IW{2,1}(15,:)'"/1 -> dotprod15/1
  dotprod14/1 -> Mux/14
  "IW{2,1}(14,:)'"/1 -> dotprod14/1
  dotprod13/1 -> Mux/13
  "IW{2,1}(13,:)'"/1 -> dotprod13/1
  dotprod12/1 -> Mux/12
  "IW{2,1}(12,:)'"/1 -> dotprod12/1
  dotprod11/1 -> Mux/11
  "IW{2,1}(11,:)'"/1 -> dotprod11/1
  dotprod10/1 -> Mux/10
  "IW{2,1}(10,:)'"/1 -> dotprod10/1
  dotprod9/1 -> Mux/9
  "IW{2,1}(9,:)'"/1 -> dotprod9/1
  dotprod8/1 -> Mux/8
  "IW{2,1}(8,:)'"/1 -> dotprod8/1
  dotprod7/1 -> Mux/7
  "IW{2,1}(7,:)'"/1 -> dotprod7/1
  dotprod6/1 -> Mux/6
  "IW{2,1}(6,:)'"/1 -> dotprod6/1
  dotprod5/1 -> Mux/5
  "IW{2,1}(5,:)'"/1 -> dotprod5/1
  dotprod4/1 -> Mux/4
  "IW{2,1}(4,:)'"/1 -> dotprod4/1
  dotprod3/1 -> Mux/3
  "IW{2,1}(3,:)'"/1 -> dotprod3/1
  dotprod2/1 -> Mux/2
  "IW{2,1}(2,:)'"/1 -> dotprod2/1
  dotprod1/1 -> Mux/1
  "ad{2,1}"/1 -> dotprod40/2, dotprod39/2, dotprod38/2, dotprod37/2, dotprod36/2, dotprod35/2, dotprod34/2, dotprod33/2, dotprod32/2, dotprod31/2, dotprod30/2, dotprod29/2, dotprod28/2, dotprod27/2, dotprod26/2, dotprod25/2, dotprod24/2, dotprod23/2, dotprod22/2, dotprod21/2, dotprod20/2, dotprod19/2, dotprod18/2, dotprod17/2, dotprod16/2, dotprod15/2, dotprod14/2, dotprod13/2, dotprod12/2, dotprod11/2, dotprod10/2, dotprod9/2, dotprod8/2, dotprod7/2, dotprod6/2, dotprod5/2, dotprod4/2, dotprod3/2, dotprod2/2, dotprod1/2
  "IW{2,1}(1,:)'"/1 -> dotprod1/1

== system hyd_hyb_2_int_cont_Final/controller1/optimized controller/SOC upper 0.5/SOC upper 0.6/SOC upper 0.7/SOC upper 0.8/net_col_c_d_8_9/Layer 3/Delays 1 ==
  "p{3}" : Inport  PortDimensions=40
  mux : Mux  Inputs=1
  "pd{3,2}" : Outport
  wires:
  mux/1 -> "pd{3,2}"/1
  "p{3}"/1 -> mux/1

== system hyd_hyb_2_int_cont_Final/controller1/optimized controller/SOC upper 0.5/SOC upper 0.6/SOC upper 0.7/SOC upper 0.8/net_col_c_d_8_9/Layer 3/LW{3,2} ==
  "ad{3,2}" : Inport  PortDimensions=40
  "IW{3,2}(1,:)'" : Constant  Value=[-0.69911497170846826;-0.84968559473564587;0.93001417164508637;0.018202841756782048;0.76378491660665193;0.84914790052554001;-0.22866747930600972;-0.70988610283860432;-0.37369799840908985;-0.77413605436519262;-0.63667272785630602;-0.13934641013435334;-0.41405897236010791;-0.50325625051054479;1.1492329270259298;0.61933422714591557;-0.7657963304111004;-0.038376686711376902;-0.66711670279845703;-0.76082072180098936;0.17440556360546713;0.089970343924166307;-0.21834942423226728;-1.0721888491060685;-0.78210940401126205;-0.45017112518459645;0.1892988776329437;-1.0423381607025282;0.56208969326132274;-0.38660183925036612;-0.57815958836389136;-0.7345342692876411;0.93555241069437889;0.84386167904683085;0.18599157668689836;0.94138927521719373;0.11694894528843508;-0.05118440700807754;-0.51667371394154937;-0.24648808072009776]
  Mux : Mux  Inputs=1
  dotprod1 : neural/Weight Functions/dotprod
  "lz{3,2}" : Outport
  wires:
  Mux/1 -> "lz{3,2}"/1
  dotprod1/1 -> Mux/1
  "ad{3,2}"/1 -> dotprod1/2
  "IW{3,2}(1,:)'"/1 -> dotprod1/1

== system hyd_hyb_2_int_cont_Final/controller1/optimized controller/SOC upper 0.5/SOC upper 0.6/SOC upper 0.7/SOC upper 0.8/net_col_e_f_8_9/Layer 1/Delays 1 ==
  "p{1}" : Inport  PortDimensions=2
  mux : Mux  Inputs=1
  "pd{1,1}" : Outport
  wires:
  mux/1 -> "pd{1,1}"/1
  "p{1}"/1 -> mux/1

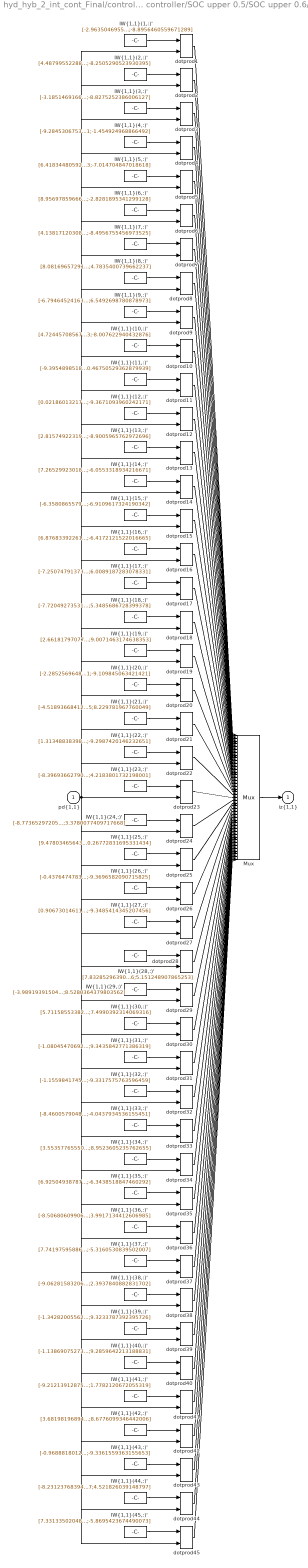
== system hyd_hyb_2_int_cont_Final/controller1/optimized controller/SOC upper 0.5/SOC upper 0.6/SOC upper 0.7/SOC upper 0.8/net_col_e_f_8_9/Layer 1/IW{1,1} ==
  "pd{1,1}" : Inport  PortDimensions=2
  "IW{1,1}(1,:)'" : Constant  Value=[-2.9635046955034552;-8.8956460559671289]
  "IW{1,1}(10,:)'" : Constant  Value=[4.724457085676093;-8.007622940432876]
  "IW{1,1}(11,:)'" : Constant  Value=[-9.3954898518962011;0.46750529362879939]
  "IW{1,1}(12,:)'" : Constant  Value=[0.021860132171899381;-9.3671093960242171]
  "IW{1,1}(13,:)'" : Constant  Value=[2.8157492231915131;-8.9005965762972696]
  "IW{1,1}(14,:)'" : Constant  Value=[7.2652992301803652;-6.0553318934216671]
  "IW{1,1}(15,:)'" : Constant  Value=[-6.3580865579587105;-6.9109617324190342]
  "IW{1,1}(16,:)'" : Constant  Value=[6.8768339226155248;-6.4172121522016665]
  "IW{1,1}(17,:)'" : Constant  Value=[-7.2507479137365545;6.0089187283078331]
  "IW{1,1}(18,:)'" : Constant  Value=[-7.7204927353107333;5.3485686728399378]
  "IW{1,1}(19,:)'" : Constant  Value=[2.6618179707793499;9.0071463174638353]
  "IW{1,1}(2,:)'" : Constant  Value=[4.4879955228817998;-8.2505290523930395]
  "IW{1,1}(20,:)'" : Constant  Value=[-2.2852569648813601;-9.109845063421421]
  "IW{1,1}(21,:)'" : Constant  Value=[-4.5189366841203045;8.229781967760049]
  "IW{1,1}(22,:)'" : Constant  Value=[1.3134883839878417;-9.2987420146232651]
  "IW{1,1}(23,:)'" : Constant  Value=[-8.3969366279041839;4.2183801732198001]
  "IW{1,1}(24,:)'" : Constant  Value=[-8.7736529720567393;3.3780077409717668]
  "IW{1,1}(25,:)'" : Constant  Value=[9.478034656431058;0.26772831695331434]
  "IW{1,1}(26,:)'" : Constant  Value=[-0.43764747837830054;-9.3696582090715825]
  "IW{1,1}(27,:)'" : Constant  Value=[0.90673014611835079;-9.3485414345207456]
  "IW{1,1}(28,:)'" : Constant  Value=[7.8328529639006366;5.151248907865253]
  "IW{1,1}(29,:)'" : Constant  Value=[-3.9891939150468474;8.5280364379803562]
  "IW{1,1}(3,:)'" : Constant  Value=[-3.1851469166119291;-8.8275252386006127]
  "IW{1,1}(30,:)'" : Constant  Value=[5.7115855338208394;7.4990392314069316]
  "IW{1,1}(31,:)'" : Constant  Value=[-1.08045470692294;9.3435842771386319]
  "IW{1,1}(32,:)'" : Constant  Value=[-1.1559841745958797;-9.3317575763596459]
  "IW{1,1}(33,:)'" : Constant  Value=[-8.4600579048837261;-4.0437934536155451]
  "IW{1,1}(34,:)'" : Constant  Value=[3.5535776555091059;8.9523605235762655]
  "IW{1,1}(35,:)'" : Constant  Value=[6.9250493878763884;-6.3438518847460292]
  "IW{1,1}(36,:)'" : Constant  Value=[-8.506806099064276;3.9917134412606985]
  "IW{1,1}(37,:)'" : Constant  Value=[7.7419759588681032;-5.3160530839502007]
  "IW{1,1}(38,:)'" : Constant  Value=[-9.0628158320699725;2.3937840882831702]
  "IW{1,1}(39,:)'" : Constant  Value=[-1.3428200556209264;9.3233787392395726]
  "IW{1,1}(4,:)'" : Constant  Value=[-9.2845306753317391;-1.454924968866492]
  "IW{1,1}(40,:)'" : Constant  Value=[-1.1386907527325472;9.2859642213188831]
  "IW{1,1}(41,:)'" : Constant  Value=[-9.2121391287506409;1.7782120672055319]
  "IW{1,1}(42,:)'" : Constant  Value=[3.6819819689433504;8.6776099346442006]
  "IW{1,1}(43,:)'" : Constant  Value=[-0.96888180126800738;-9.3361559363155653]
  "IW{1,1}(44,:)'" : Constant  Value=[-8.2312376839432737;4.521826039148797]
  "IW{1,1}(45,:)'" : Constant  Value=[7.3313350204841488;-5.8695423674490073]
  "IW{1,1}(5,:)'" : Constant  Value=[6.4183448059220893;-7.014704847018618]
  "IW{1,1}(6,:)'" : Constant  Value=[8.9569785966681223;-2.8281895341299128]
  "IW{1,1}(7,:)'" : Constant  Value=[4.1381712030864835;-8.4956755456973525]
  "IW{1,1}(8,:)'" : Constant  Value=[8.0816965729149359;4.7835400739662237]
  "IW{1,1}(9,:)'" : Constant  Value=[-6.7946452416305378;6.5492698780878973]
  Mux : Mux  Inputs=45
  dotprod{1..45} (45 alike) : neural/Weight Functions/dotprod
  "iz{1,1}" : Outport
  wires:
  Mux/1 -> "iz{1,1}"/1
  dotprod45/1 -> Mux/45
  "IW{1,1}(45,:)'"/1 -> dotprod45/1
  dotprod44/1 -> Mux/44
  "IW{1,1}(44,:)'"/1 -> dotprod44/1
  dotprod43/1 -> Mux/43
  "IW{1,1}(43,:)'"/1 -> dotprod43/1
  dotprod42/1 -> Mux/42
  "IW{1,1}(42,:)'"/1 -> dotprod42/1
  dotprod41/1 -> Mux/41
  "IW{1,1}(41,:)'"/1 -> dotprod41/1
  dotprod40/1 -> Mux/40
  "IW{1,1}(40,:)'"/1 -> dotprod40/1
  dotprod39/1 -> Mux/39
  "IW{1,1}(39,:)'"/1 -> dotprod39/1
  dotprod38/1 -> Mux/38
  "IW{1,1}(38,:)'"/1 -> dotprod38/1
  dotprod37/1 -> Mux/37
  "IW{1,1}(37,:)'"/1 -> dotprod37/1
  dotprod36/1 -> Mux/36
  "IW{1,1}(36,:)'"/1 -> dotprod36/1
  dotprod35/1 -> Mux/35
  "IW{1,1}(35,:)'"/1 -> dotprod35/1
  dotprod34/1 -> Mux/34
  "IW{1,1}(34,:)'"/1 -> dotprod34/1
  dotprod33/1 -> Mux/33
  "IW{1,1}(33,:)'"/1 -> dotprod33/1
  dotprod32/1 -> Mux/32
  "IW{1,1}(32,:)'"/1 -> dotprod32/1
  dotprod31/1 -> Mux/31
  "IW{1,1}(31,:)'"/1 -> dotprod31/1
  dotprod30/1 -> Mux/30
  "IW{1,1}(30,:)'"/1 -> dotprod30/1
  dotprod29/1 -> Mux/29
  "IW{1,1}(29,:)'"/1 -> dotprod29/1
  dotprod28/1 -> Mux/28
  "IW{1,1}(28,:)'"/1 -> dotprod28/1
  dotprod27/1 -> Mux/27
  "IW{1,1}(27,:)'"/1 -> dotprod27/1
  dotprod26/1 -> Mux/26
  "IW{1,1}(26,:)'"/1 -> dotprod26/1
  dotprod25/1 -> Mux/25
  "IW{1,1}(25,:)'"/1 -> dotprod25/1
  dotprod24/1 -> Mux/24
  "IW{1,1}(24,:)'"/1 -> dotprod24/1
  dotprod23/1 -> Mux/23
  "IW{1,1}(23,:)'"/1 -> dotprod23/1
  dotprod22/1 -> Mux/22
  "IW{1,1}(22,:)'"/1 -> dotprod22/1
  dotprod21/1 -> Mux/21
  "IW{1,1}(21,:)'"/1 -> dotprod21/1
  dotprod20/1 -> Mux/20
  "IW{1,1}(20,:)'"/1 -> dotprod20/1
  dotprod19/1 -> Mux/19
  "IW{1,1}(19,:)'"/1 -> dotprod19/1
  dotprod18/1 -> Mux/18
  "IW{1,1}(18,:)'"/1 -> dotprod18/1
  dotprod17/1 -> Mux/17
  "IW{1,1}(17,:)'"/1 -> dotprod17/1
  dotprod16/1 -> Mux/16
  "IW{1,1}(16,:)'"/1 -> dotprod16/1
  dotprod15/1 -> Mux/15
  "IW{1,1}(15,:)'"/1 -> dotprod15/1
  dotprod14/1 -> Mux/14
  "IW{1,1}(14,:)'"/1 -> dotprod14/1
  dotprod13/1 -> Mux/13
  "IW{1,1}(13,:)'"/1 -> dotprod13/1
  dotprod12/1 -> Mux/12
  "IW{1,1}(12,:)'"/1 -> dotprod12/1
  dotprod11/1 -> Mux/11
  "IW{1,1}(11,:)'"/1 -> dotprod11/1
  dotprod10/1 -> Mux/10
  "IW{1,1}(10,:)'"/1 -> dotprod10/1
  dotprod9/1 -> Mux/9
  "IW{1,1}(9,:)'"/1 -> dotprod9/1
  dotprod8/1 -> Mux/8
  "IW{1,1}(8,:)'"/1 -> dotprod8/1
  dotprod7/1 -> Mux/7
  "IW{1,1}(7,:)'"/1 -> dotprod7/1
  dotprod6/1 -> Mux/6
  "IW{1,1}(6,:)'"/1 -> dotprod6/1
  dotprod5/1 -> Mux/5
  "IW{1,1}(5,:)'"/1 -> dotprod5/1
  dotprod4/1 -> Mux/4
  "IW{1,1}(4,:)'"/1 -> dotprod4/1
  dotprod3/1 -> Mux/3
  "IW{1,1}(3,:)'"/1 -> dotprod3/1
  dotprod2/1 -> Mux/2
  "IW{1,1}(2,:)'"/1 -> dotprod2/1
  dotprod1/1 -> Mux/1
  "pd{1,1}"/1 -> dotprod45/2, dotprod44/2, dotprod43/2, dotprod42/2, dotprod41/2, dotprod40/2, dotprod39/2, dotprod38/2, dotprod37/2, dotprod36/2, dotprod35/2, dotprod34/2, dotprod33/2, dotprod32/2, dotprod31/2, dotprod30/2, dotprod29/2, dotprod28/2, dotprod27/2, dotprod26/2, dotprod25/2, dotprod24/2, dotprod23/2, dotprod22/2, dotprod21/2, dotprod20/2, dotprod19/2, dotprod18/2, dotprod17/2, dotprod16/2, dotprod15/2, dotprod14/2, dotprod13/2, dotprod12/2, dotprod11/2, dotprod10/2, dotprod9/2, dotprod8/2, dotprod7/2, dotprod6/2, dotprod5/2, dotprod4/2, dotprod3/2, dotprod2/2, dotprod1/2
  "IW{1,1}(1,:)'"/1 -> dotprod1/1

== system hyd_hyb_2_int_cont_Final/controller1/optimized controller/SOC upper 0.5/SOC upper 0.6/SOC upper 0.7/SOC upper 0.8/net_col_e_f_8_9/Layer 2/Delays 1 ==
  "p{2}" : Inport  PortDimensions=45
  mux : Mux  Inputs=1
  "pd{2,1}" : Outport
  wires:
  mux/1 -> "pd{2,1}"/1
  "p{2}"/1 -> mux/1
